simulink model "sensor_GPS_model"  (R2025b)
settings: Solver=FixedStepDiscrete  StartTime=0.0  StopTime=20  FixedStep=0.001  RelTol=1e-3
values from neighbouring files (symbols this model uses):
  GPS_POS_H_NOISE = 0.5    [SensorDict.sldd]
  GPS_POS_V_NOISE = 1.0    [SensorDict.sldd]
  GPS_SAMPLE_RATE = 5.0    [SensorDict.sldd]
  GPS_VEL_NOISE = 0.1    [SensorDict.sldd]
libraries: simulink x4
settings Model: DataDictionary=SensorDict.sldd  Creator=89447  LastModifiedBy=89447

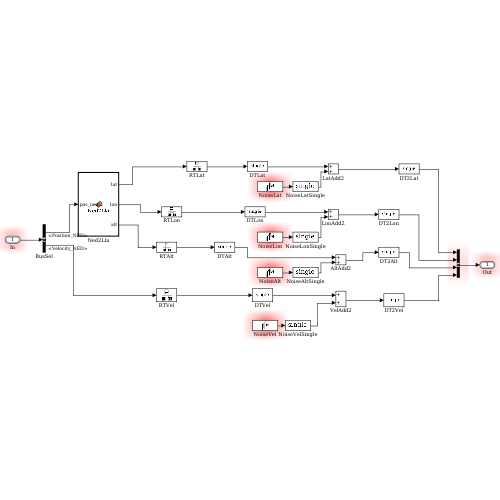
[thumbnail: Simulink's stored preview of the top-level diagram]
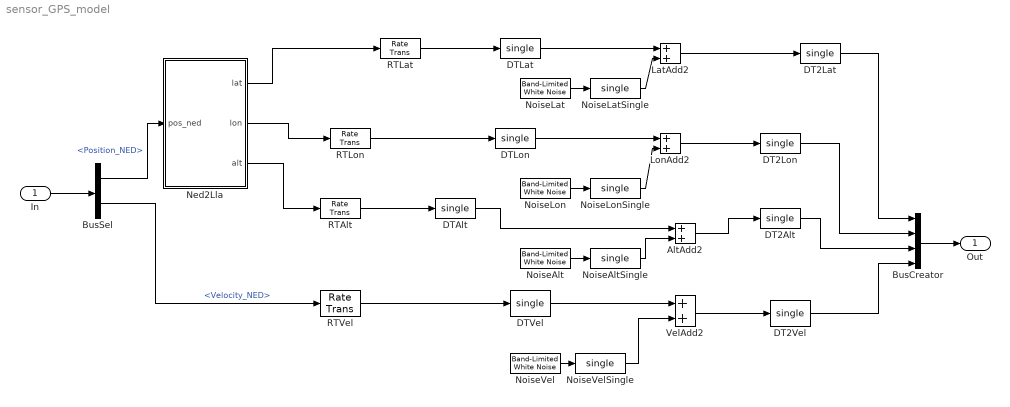
== system sensor_GPS_model ==
  In : Inport  OutDataTypeStr=Bus: DynamicModelBus
  AltAdd2 : Sum
  BusCreator : BusCreator  Inputs=4  OutDataTypeStr=Bus: GPS_BUS  NonVirtualBus=on
      settings: InheritFromInputs=off
  BusSel : BusSelector  OutputSignals=Position_NED,Velocity_NED
  DT2Alt : DataTypeConversion  OutDataTypeStr=single  SaturateOnIntegerOverflow=off  RndMeth=Floor
  DT2Lat : DataTypeConversion  OutDataTypeStr=single  SaturateOnIntegerOverflow=off  RndMeth=Floor
  DT2Lon : DataTypeConversion  OutDataTypeStr=single  SaturateOnIntegerOverflow=off  RndMeth=Floor
  DT2Vel : DataTypeConversion  OutDataTypeStr=single  SaturateOnIntegerOverflow=off  RndMeth=Floor
  DTAlt : DataTypeConversion  OutDataTypeStr=single  SaturateOnIntegerOverflow=off  RndMeth=Floor
  DTLat : DataTypeConversion  OutDataTypeStr=single  SaturateOnIntegerOverflow=off  RndMeth=Floor
  DTLon : DataTypeConversion  OutDataTypeStr=single  SaturateOnIntegerOverflow=off  RndMeth=Floor
  DTVel : DataTypeConversion  OutDataTypeStr=single  SaturateOnIntegerOverflow=off  RndMeth=Floor
  LatAdd2 : Sum
  LonAdd2 : Sum
  Ned2Lla : MATLAB Function  TreatAsAtomicUnit=on
  NoiseAlt : simulink/Sources/Band-Limited White Noise  Cov=GPS_POS_V_NOISE^2 / GPS_SAMPLE_RATE  Ts=1 / double(GPS_SAMPLE_RATE)  seed=45603
  NoiseAltSingle : DataTypeConversion  OutDataTypeStr=single  SaturateOnIntegerOverflow=off  RndMeth=Floor
  NoiseLat : simulink/Sources/Band-Limited White Noise  Cov=GPS_POS_H_NOISE^2 / GPS_SAMPLE_RATE  Ts=1 / double(GPS_SAMPLE_RATE)  seed=45601
  NoiseLatSingle : DataTypeConversion  OutDataTypeStr=single  SaturateOnIntegerOverflow=off  RndMeth=Floor
  NoiseLon : simulink/Sources/Band-Limited White Noise  Cov=GPS_POS_H_NOISE^2 / GPS_SAMPLE_RATE  Ts=1 / double(GPS_SAMPLE_RATE)  seed=45602
  NoiseLonSingle : DataTypeConversion  OutDataTypeStr=single  SaturateOnIntegerOverflow=off  RndMeth=Floor
  NoiseVel : simulink/Sources/Band-Limited White Noise  Cov=GPS_VEL_NOISE^2 / GPS_SAMPLE_RATE  Ts=1 / double(GPS_SAMPLE_RATE)  seed=45604
  NoiseVelSingle : DataTypeConversion  OutDataTypeStr=single  SaturateOnIntegerOverflow=off  RndMeth=Floor
  RTAlt : RateTransition
  RTLat : RateTransition
  RTLon : RateTransition
  RTVel : RateTransition
  VelAdd2 : Sum
  Out : Outport  OutDataTypeStr=Bus: GPS_BUS
  wires:
  In/1 -> BusSel/1
  BusSel/1 -> Ned2Lla/1(pos_ned)  "<Position_NED>"
  BusCreator/1 -> Out/1
  RTLat/1 -> DTLat/1
  RTLon/1 -> DTLon/1
  RTAlt/1 -> DTAlt/1
  RTVel/1 -> DTVel/1
  DTLat/1 -> LatAdd2/1
  DTLon/1 -> LonAdd2/1
  DTAlt/1 -> AltAdd2/1
  DTVel/1 -> VelAdd2/1
  Ned2Lla/1(lat) -> RTLat/1
  Ned2Lla/2(lon) -> RTLon/1
  Ned2Lla/3(alt) -> RTAlt/1
  BusSel/2 -> RTVel/1  "<Velocity_NED>"
  LatAdd2/1 -> DT2Lat/1
  LonAdd2/1 -> DT2Lon/1
  AltAdd2/1 -> DT2Alt/1
  VelAdd2/1 -> DT2Vel/1
  DT2Lat/1 -> BusCreator/1
  DT2Lon/1 -> BusCreator/2
  DT2Alt/1 -> BusCreator/3
  DT2Vel/1 -> BusCreator/4
  NoiseLat/1 -> NoiseLatSingle/1
  NoiseLatSingle/1 -> LatAdd2/2
  NoiseLon/1 -> NoiseLonSingle/1
  NoiseLonSingle/1 -> LonAdd2/2
  NoiseAlt/1 -> NoiseAltSingle/1
  NoiseAltSingle/1 -> AltAdd2/2
  NoiseVel/1 -> NoiseVelSingle/1
  NoiseVelSingle/1 -> VelAdd2/2

== matlab function sensor_GPS_model/Ned2Lla ==
  data: pos_ned input; lat output; lon output; alt output
function [lat, lon, alt] = Ned2Lla(pos_ned)
%#codegen
% Ned2Lla: NED位置(m) -> LLA(deg, deg, m)
% 使用球面近似, 参考点由 GPS_REF_LAT/GPS_REF_LON 定义
% pos_ned: [N, E, D] (m), single
% lat/lon: deg, alt: m (高度, -D)

R_earth = single(6371000);  % 地球半径(m)
lat_ref = single(0.0);     % GPS_REF_LAT (deg)
lon_ref = single(10.0);    % GPS_REF_LON (deg)
deg2rad_val = single(pi/180);
rad2deg_val = single(180/pi);

north = pos_ned(1);
east  = pos_ned(2);
down  = pos_ned(3);

% 纬度: lat = lat_ref + north/R * (180/pi)
lat = lat_ref + (north / R_earth) * rad2deg_val;

% 经度: lon = lon_ref + east/(R*cos(lat_ref)) * (180/pi)
cos_lat = cos(lat_ref * deg2rad_val);
lon = lon_ref + (east / (R_earth * cos_lat)) * rad2deg_val;

% 高度: alt = -down (NED中down为正)
alt = -down;
end
